simulink model "HL_control_pos_FFforce_RC_WirtualWall_Sync"  (R2020a)
settings: Solver=ode4  StartTime=0.0  StopTime=inf  FixedStep=0.001  RelTol=1e-3
libraries: xpcethercatlib x42, simulink x12, slrtlib x10, AssistOn_Gait_Lib x6
(part 1 of 3)
settings Model: xpc_rtwmakecfg_data=_xpcethercatlib_  SimulationMode=external  Creator=AliYasar  LastModifiedBy=AssistON-Gait
settings DataIOCC: SaveFormat=StructureWithTime
settings OptimizationCC: BlockReduction=off  OptimizeBlockIOStorage=off  BufferReuse=off  GlobalBufferReuse=off  ExpressionFolding=off  LocalBlockOutputs=off  OptimizeDataStoreBuffers=off  BusAssignmentInplaceUpdate=off
settings HardwareCC: ProdBitPerPointer=32  ProdBitPerSizeT=32  ProdBitPerPtrDiffT=32  ProdLargestAtomicFloat=None  ProdWordSize=32  ProdLongLongMode=on  ProdHWDeviceType=Generic->32-bit x86 compatible
settings RTWCC: Description=Simulink Real-Time  SystemTargetFile=slrt.tlc  TemplateMakefile=slrt_default_tmf  CodeExecutionProfiling=on  RTWCompilerOptimization=on
settings SimulinkRealTimeCC: SupportVariableSizeSignals=on  RL32LogTETModifier=off  xPCConcurrentTasks=on  xPCEnableSFAnimation=on

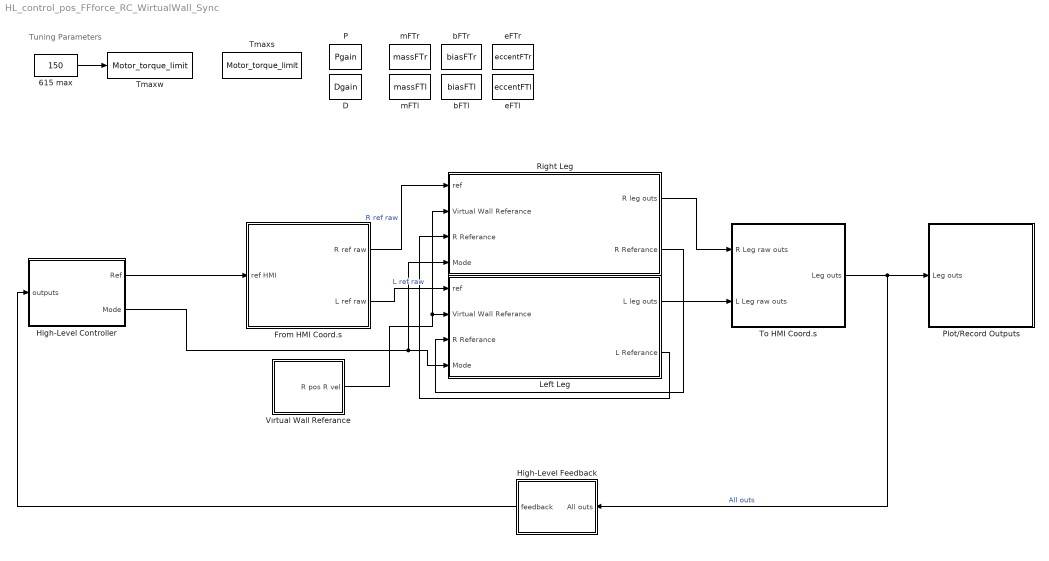
== system HL_control_pos_FFforce_RC_WirtualWall_Sync ==
  note: Tuning Parameters
  615 max : Constant  Value=150
  D : DataStoreMemory  DataStoreName=Dgain  ReadBeforeWriteMsg=warning  WriteAfterWriteMsg=warning  WriteAfterReadMsg=warning  ShowAdditionalParam=off  OutDataTypeStr=double  Dimensions=1
      settings: RTWStateStorageClass=ExportedGlobal
  From HMI Coord.s : Subsystem
  High-Level Controller : Subsystem
  High-Level Feedback : Subsystem
  Left Leg : Subsystem
  P : DataStoreMemory  DataStoreName=Pgain  ReadBeforeWriteMsg=warning  WriteAfterWriteMsg=warning  WriteAfterReadMsg=warning  ShowAdditionalParam=off  OutDataTypeStr=double  Dimensions=1
      settings: RTWStateStorageClass=ExportedGlobal
  Plot/Record Outputs : Subsystem
  Right Leg : Subsystem
  Tmaxs : DataStoreMemory  DataStoreName=Motor_torque_limit  ReadBeforeWriteMsg=warning  WriteAfterWriteMsg=warning  WriteAfterReadMsg=warning  ShowAdditionalParam=off  OutDataTypeStr=double
  Tmaxw : DataStoreWrite  DataStoreName=Motor_torque_limit
  To HMI Coord.s : Subsystem
  Vırtual Wall Referance : Subsystem
  bFTl : DataStoreMemory  DataStoreName=biasFTl  ReadBeforeWriteMsg=warning  WriteAfterWriteMsg=warning  WriteAfterReadMsg=warning  InitialValue=[0; 0; 0; 0; 0; 0]  ShowAdditionalParam=off  OutDataTypeStr=double  Dimensions=[6 1]
      settings: RTWStateStorageClass=ExportedGlobal
  bFTr : DataStoreMemory  DataStoreName=biasFTr  ReadBeforeWriteMsg=warning  WriteAfterWriteMsg=warning  WriteAfterReadMsg=warning  InitialValue=[0; 0; 0; 0; 0; 0]  ShowAdditionalParam=off  OutDataTypeStr=double  Dimensions=[6 1]
      settings: RTWStateStorageClass=ExportedGlobal
  eFTl : DataStoreMemory  DataStoreName=eccentFTl  ReadBeforeWriteMsg=warning  WriteAfterWriteMsg=warning  WriteAfterReadMsg=warning  InitialValue=[0; 0; 0]  ShowAdditionalParam=off  OutDataTypeStr=double  Dimensions=[3 1]
      settings: RTWStateStorageClass=ExportedGlobal
  eFTr : DataStoreMemory  DataStoreName=eccentFTr  ReadBeforeWriteMsg=warning  WriteAfterWriteMsg=warning  WriteAfterReadMsg=warning  InitialValue=[0; 0; 0]  ShowAdditionalParam=off  OutDataTypeStr=double  Dimensions=[3 1]
      settings: RTWStateStorageClass=ExportedGlobal
  mFTl : DataStoreMemory  DataStoreName=massFTl  ReadBeforeWriteMsg=warning  WriteAfterWriteMsg=warning  WriteAfterReadMsg=warning  ShowAdditionalParam=off  OutDataTypeStr=double  Dimensions=1
      settings: RTWStateStorageClass=ExportedGlobal
  mFTr : DataStoreMemory  DataStoreName=massFTr  ReadBeforeWriteMsg=warning  WriteAfterWriteMsg=warning  WriteAfterReadMsg=warning  ShowAdditionalParam=off  OutDataTypeStr=double  Dimensions=1
      settings: RTWStateStorageClass=ExportedGlobal
  wires:
  615 max/1 -> Tmaxw/1
  Left Leg/1(L leg outs) -> To HMI Coord.s/2(L Leg raw outs)
  Right Leg/1(R leg outs) -> To HMI Coord.s/1(R Leg raw outs)
  To HMI Coord.s/1(Leg outs) -> High-Level Feedback/1(All outs), Plot/Record Outputs/1(Leg outs)  "All outs"
  High-Level Controller/1(Ref) -> From HMI Coord.s/1(ref HMI)
  From HMI Coord.s/2(L ref raw) -> Left Leg/1(ref)  "L ref raw"
  From HMI Coord.s/1(R ref raw) -> Right Leg/1(ref)  "R ref raw"
  High-Level Feedback/1(feedback) -> High-Level Controller/1(outputs)
  Right Leg/2(R Referance) -> Left Leg/3(R Referance)
  Left Leg/2(L Referance) -> Right Leg/3("R Referance ")
  Vırtual Wall Referance/1(R pos R vel) -> Left Leg/2(Virtual Wall Referance), Right Leg/2(Virtual Wall Referance)
  High-Level Controller/2(Mode) -> Right Leg/4(Mode), Left Leg/4(Mode)

== system HL_control_pos_FFforce_RC_WirtualWall_Sync/From HMI Coord.s ==
  ref HMI : Inport
  Anti-gravity force : Constant  Value=0
  Bus Selector : BusSelector  OutputSignals=right,left
  "N.m -> mN.m" : Gain  Gain=1000
  Reference : Subsystem
  Subject mass : Constant  Value=0
  Transform L Hip to HMI Coord.s : Subsystem
  Transform R Hip to HMI Coord.s : Subsystem
  R ref raw : Outport
  L ref raw : Outport  Port=2
  wires:
  Transform R Hip to HMI Coord.s/1(R ref raw) -> R ref raw/1  "R ref raw"
  Transform L Hip to HMI Coord.s/1(L ref raw) -> L ref raw/1  "L ref raw"
  Bus Selector/1 -> Transform R Hip to HMI Coord.s/1(R ref HMI)  "<right>"
  Bus Selector/2 -> Transform L Hip to HMI Coord.s/2(L ref HMI)  "<left>"
  Subject mass/1 -> "N.m -> mN.m"/1
  ref HMI/1 -> Reference/1(HMI ref), Bus Selector/1  "HMI ref"
  "N.m -> mN.m"/1 -> Transform L Hip to HMI Coord.s/1(T scale), Transform R Hip to HMI Coord.s/2(T scale)
  Anti-gravity force/1 -> Transform L Hip to HMI Coord.s/3(In3), Transform R Hip to HMI Coord.s/3(In3)

== system HL_control_pos_FFforce_RC_WirtualWall_Sync/High-Level Controller ==
  outputs : Inport
  Home Position: 0 Calibration: 1 Force Control w/ FSR: 2 Power OFF: any : Constant  Value=0
  Reference Generator : Stateflow chart  TreatAsAtomicUnit=on
      settings: PortSchema="{\"entries\":[{\"content\":{\"sides\":[{\"content\":{\"connectorIds\":[\"In1\",\"In4\",\"In2\",\"In3\"]},\"type\":\"ConnectorPlacement.EquallySpacedRectSide\",\"uuid\":\"aa4ba9cf-5d9b-4aac-b6bf-f3c223218dd1\"},{\"content\":{\"connectorIds\":[\"Out1\"],\"side\":\"RIGHT\"},\"type\":\"ConnectorPlacement.EquallySpacedRectSide\",\"uuid\":\"cd1fa299-8856-4d1c-b1a3-02aa84ed53a9\"},{\"content\":{\"connectorIds\":[\"In5\"],\"side\":\"TOP\"},\"type\":\"ConnectorPlacement.EquallySpacedRectSide\",\"uuid\":\"78c29b93-9a46-49f0-9d97-93372759fd65\"}]},\"type\":\"ConnectorPlacement.EquallySpacedConnector\",\"uuid\":\"ad73f022-92f1-404d-a46a-c53ca5f2e508\"}],\"packageUris\":[\"http://schema.mathworks.com/mf0/Connector/19700101\"],\"version\":\"1.0\"}"
  Select outputs : Subsystem
  System Enable : Stateflow chart  TreatAsAtomicUnit=on
      settings: PortSchema="{\"entries\":[{\"content\":{\"sides\":[{\"content\":{\"connectorIds\":[\"In2\",\"In1\"]},\"type\":\"ConnectorPlacement.EquallySpacedRectSide\",\"uuid\":\"4b9d4f11-1327-467a-8cb8-f29f037cc139\"},{\"content\":{\"connectorIds\":[\"Out2\",\"Out1\"],\"side\":\"RIGHT\"},\"type\":\"ConnectorPlacement.EquallySpacedRectSide\",\"uuid\":\"fda62fdb-ec88-4c1e-8450-5399b215f716\"},{\"content\":{\"connectorIds\":[],\"side\":\"TOP\"},\"type\":\"ConnectorPlacement.EquallySpacedRectSide\",\"uuid\":\"5cb4c28a-5e87-4a76-a578-be8042483ab0\"}]},\"type\":\"ConnectorPlacement.EquallySpacedConnector\",\"uuid\":\"90f57a99-7211-48b6-a431-558685cd5a2d\"}],\"packageUris\":[\"http://schema.mathworks.com/mf0/Connector/19700101\"],\"version\":\"1.0\"}"
  "To clear the error, change the value to any number" : Constant
  Ref : Outport
  Mode : Outport  Port=2
  tag scope: status=global
  wires:
  Reference Generator/1(ref) -> Ref/1  "HMI ref"
  System Enable/1(sysON) -> Reference Generator/1(sysON)
  Home Position: 0 Calibration: 1 Force Control w/ FSR: 2 Power OFF: any/1 -> Reference Generator/5(MODE), Mode/1
  "To clear the error, change the value to any number"/1 -> System Enable/2(clear)
  outputs/1 -> Select outputs/1(outs)
  Select outputs/1(disk angles) -> System Enable/1(diskpos)
  Select outputs/2(gait out) -> Reference Generator/4(gait)
  Select outputs/3(FT out) -> Reference Generator/2(FT)
  Select outputs/4(EE mot) -> Reference Generator/3(mot)
  System Enable/2(stat) -> [status]

== system HL_control_pos_FFforce_RC_WirtualWall_Sync/High-Level Feedback ==
  All outs : Inport
  Bus Creator : BusCreator  Inputs=3
  Bus Creator1 : BusCreator  Inputs=2  OutDataTypeStr=Bus: HeelForce
      settings: InheritFromInputs=off
  Bus Selector : BusSelector  OutputSignals=R Leg outs.R_foot_sens,L Leg outs.L_foot_sens,R Leg outs,L Leg outs
  Heel Sensor : Stateflow chart  TreatAsAtomicUnit=on
  feedback : Outport
  wires:
  Bus Creator/1 -> feedback/1
  Heel Sensor/1(gait) -> Bus Creator/1
  Bus Selector/2 -> Bus Creator1/2  "<L_foot_sens>"
  Bus Selector/4 -> Bus Creator/3  "<L Leg outs>"
  Bus Creator1/1 -> Heel Sensor/1(heel_force)
  Bus Selector/1 -> Bus Creator1/1  "<R_foot_sens>"
  Bus Selector/3 -> Bus Creator/2  "<R Leg outs>"
  All outs/1 -> Bus Selector/1

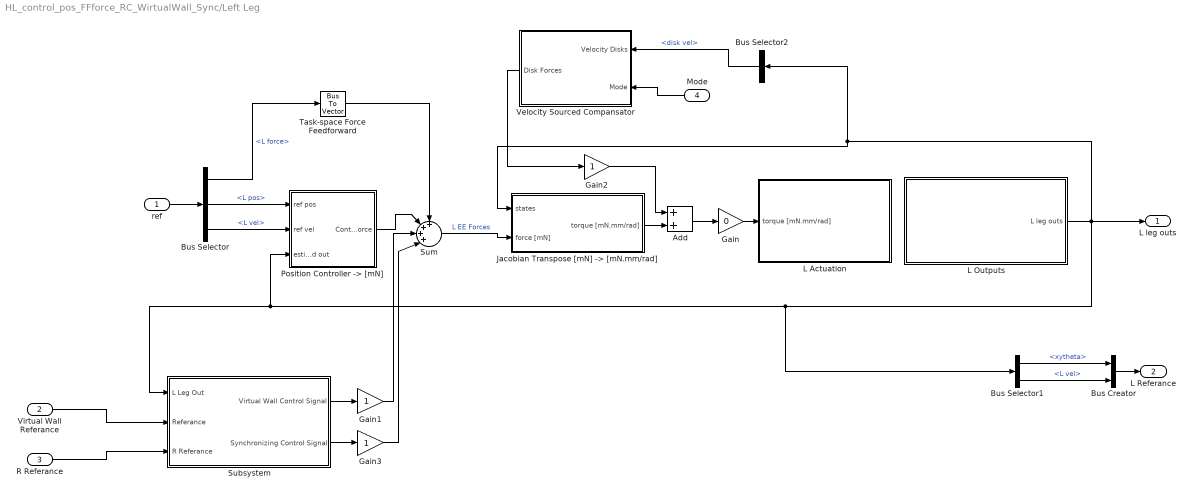
== system HL_control_pos_FFforce_RC_WirtualWall_Sync/Left Leg ==
  ref : Inport
  Virtual Wall Referance : Inport  Port=2
  R Referance : Inport  Port=3
  Mode : Inport  Port=4
  Add : Sum
  Bus Creator : BusCreator  Inputs=2
  Bus Selector : BusSelector  OutputSignals=L force,L pos,L vel
  Bus Selector1 : BusSelector  OutputSignals=L pos.xytheta,L vel
  Bus Selector2 : BusSelector  OutputSignals=L disk mot.disk vel
  Gain : Gain  Gain=0
  Gain1 : Gain
  Gain2 : Gain
  Gain3 : Gain
  "Jacobian Transpose [mN] -> [mN.mm/rad]" : Subsystem
  L Actuation : Subsystem
  L Outputs : Subsystem
  "Position Controller -> [mN]" : Subsystem
  Subsystem : Subsystem
  Sum : Sum  Inputs=++++|
  Task-space Force Feedforward : BusToVector
  Velocity Sourced Compansator : Subsystem
  L leg outs : Outport
  L Referance : Outport  Port=2
  wires:
  Task-space Force Feedforward/1 -> Sum/1
  Gain/1 -> L Actuation/1(torque [mN.mm/rad])
  ref/1 -> Bus Selector/1
  Bus Selector/2 -> "Position Controller -> [mN]"/1(ref pos)  "<L pos>"
  Bus Selector/1 -> Task-space Force Feedforward/1  "<L force>"
  "Position Controller -> [mN]"/1(Control Force) -> Sum/2
  Sum/1 -> "Jacobian Transpose [mN] -> [mN.mm/rad]"/2(force [mN])  "L EE Forces"
  Bus Selector/3 -> "Position Controller -> [mN]"/2(ref vel)  "<L vel>"
  Bus Selector1/1 -> Bus Creator/1  "<xytheta>"
  Bus Selector1/2 -> Bus Creator/2  "<L vel>"
  Bus Creator/1 -> L Referance/1
  L Outputs/1(L leg outs) -> Bus Selector1/1, Subsystem/1(L Leg Out), "Position Controller -> [mN]"/3(estimated out), Bus Selector2/1, "Jacobian Transpose [mN] -> [mN.mm/rad]"/1(states), L leg outs/1
  Mode/1 -> Velocity Sourced Compansator/2(Mode)
  Bus Selector2/1 -> Velocity Sourced Compansator/1(Velocity Disks)  "<disk vel>"
  "Jacobian Transpose [mN] -> [mN.mm/rad]"/1(torque [mN.mm/rad]) -> Add/2
  Add/1 -> Gain/1
  Velocity Sourced Compansator/1(Disk Forces) -> Gain2/1
  Gain2/1 -> Add/1
  Virtual Wall Referance/1 -> Subsystem/2(Referance)
  R Referance/1 -> Subsystem/3(R Referance)
  Subsystem/1(Virtual Wall Control Signal) -> Gain1/1
  Subsystem/2(Synchronizing Control Signal) -> Gain3/1
  Gain1/1 -> Sum/3
  Gain3/1 -> Sum/4

== system HL_control_pos_FFforce_RC_WirtualWall_Sync/Plot//Record Outputs ==
  Leg outs : Inport
  Bus Creator2 : BusCreator  Inputs=3
  Bus Selector1 : BusSelector  OutputSignals=R Leg outs.rFT.rFx,R Leg outs.rFT.rFy,R Leg outs.rFT.rTx,R Leg outs.rFT.rTy,R Leg outs.rFT.rTz,L Leg outs.lFT.lFx,L Leg outs.lFT.lFy,L Leg outs.lFT.lTx,L Leg outs.lFT.lTy,L Leg outs.lFT.lTz  OutputAsBus=on
  Bus Selector3 : BusSelector  OutputSignals=R Leg outs.R Motor Torques,L Leg outs.L Motor Torques  OutputAsBus=on
  Bus Selector4 : BusSelector  OutputSignals=R Leg outs.R_foot_sens,L Leg outs.L_foot_sens  OutputAsBus=on
  Bus Selector5 : BusSelector  OutputSignals=R Leg outs,L Leg outs
  FT Readings : slrtlib/Displays and Logging/Scope   scopeno=12  scopetype=Target  autostart=on  viewmode=Numerical  formatstr='%15.6f'  grid=on  ylimits=100*[-1, 1]  nosamples=10  noprepostsamples=0  interleave=10  triggermode=FreeRun  triggersignal=1  trigsignalfromport=off  triggerlevel=0.0  triggerslope=Either  triggerscope=1  triggersample=0  filename=data.dat  mode=Lazy  writesize=512  autorestart=off  dynamicfilemode=off  maxwritefilesize=512*1024^2
  Heel Strikes : slrtlib/Displays and Logging/Scope   scopeno=13  scopetype=Target  autostart=on  viewmode=Graphical rolling  formatstr='%15.6f'  grid=on  ylimits=5*[-0.2, 1]  nosamples=500  noprepostsamples=0  interleave=20  triggermode=FreeRun  triggersignal=1  trigsignalfromport=off  triggerlevel=0.0  triggerslope=Either  triggerscope=1  triggersample=0  filename=data.dat  mode=Lazy  writesize=512  autorestart=off  dynamicfilemode=off  maxwritefilesize=512*1024^2
  Left leg readings : Subsystem
  Motor Torque Demand : slrtlib/Displays and Logging/Scope   scopeno=11  scopetype=Target  autostart=on  viewmode=Numerical  formatstr='%15.6f'  grid=on  ylimits=100*[-1, 1]  nosamples=10  noprepostsamples=0  interleave=10  triggermode=FreeRun  triggersignal=1  trigsignalfromport=off  triggerlevel=0.0  triggerslope=Either  triggerscope=1  triggersample=0  filename=data.dat  mode=Lazy  writesize=512  autorestart=off  dynamicfilemode=off  maxwritefilesize=512*1024^2
  Right leg readings : Subsystem
  "Scope " : slrtlib/Displays and Logging/Scope   scopeno=100  scopetype=File  autostart=on  viewmode=Numerical  formatstr='%15.6f'  grid=on  ylimits=[0,0]  nosamples=100*60*60  noprepostsamples=0  interleave=10  triggermode=FreeRun  triggersignal=1  trigsignalfromport=off  triggerlevel=0.0  triggerslope=Either  triggerscope=1  triggersample=0  filename=alldata.dat  mode=Lazy  writesize=512  autorestart=off  dynamicfilemode=off  maxwritefilesize=512*1024^2
  wires:
  Bus Creator2/1 -> "Scope "/1
  Bus Selector3/1 -> Motor Torque Demand/1
  [Ref] -> Bus Creator2/2  "HMI ref"
  Bus Selector1/1 -> FT Readings/1
  Bus Selector5/2 -> Left leg readings/1(L outs)  "<L Leg outs>"
  Leg outs/1 -> Bus Selector5/1, Bus Creator2/1, Bus Selector3/1, Bus Selector4/1, Bus Selector1/1
  Bus Selector5/1 -> Right leg readings/1(R outs)  "<R Leg outs>"
  Bus Selector4/1 -> Heel Strikes/1
  [status] -> Bus Creator2/3

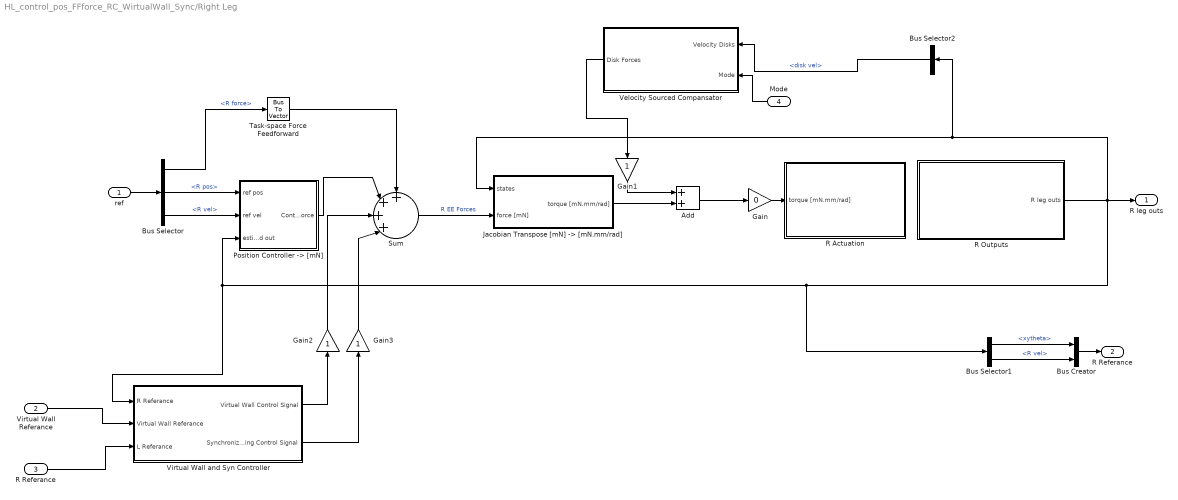
== system HL_control_pos_FFforce_RC_WirtualWall_Sync/Right Leg ==
  ref : Inport
  Virtual Wall Referance : Inport  Port=2
  "R Referance " : Inport  Port=3
  Mode : Inport  Port=4
  Add : Sum
  Bus Creator : BusCreator  Inputs=2
  Bus Selector : BusSelector  OutputSignals=R force,R pos,R vel
  Bus Selector1 : BusSelector  OutputSignals=R pos.xytheta,R vel
  Bus Selector2 : BusSelector  OutputSignals=R disk mot.disk vel
  Gain : Gain  Gain=0
  Gain1 : Gain
  Gain2 : Gain
  Gain3 : Gain
  "Jacobian Transpose [mN] -> [mN.mm/rad]" : Subsystem
  "Position Controller -> [mN]" : Subsystem
  R Actuation : Subsystem
  R Outputs : Subsystem
  Sum : Sum  Inputs=++++|
  Task-space Force Feedforward : BusToVector
  Velocity Sourced Compansator : Subsystem
  Virtual Wall and Syn Controller : Subsystem
  R leg outs : Outport
  R Referance : Outport  Port=2
  wires:
  Gain/1 -> R Actuation/1(torque [mN.mm/rad])
  Bus Selector/1 -> Task-space Force Feedforward/1  "<R force>"
  ref/1 -> Bus Selector/1
  Bus Selector/2 -> "Position Controller -> [mN]"/1(ref pos)  "<R pos>"
  Sum/1 -> "Jacobian Transpose [mN] -> [mN.mm/rad]"/2(force [mN])  "R EE Forces"
  Bus Selector/3 -> "Position Controller -> [mN]"/2(ref vel)  "<R vel>"
  Bus Creator/1 -> R Referance/1
  Bus Selector1/1 -> Bus Creator/1  "<xytheta>"
  Bus Selector1/2 -> Bus Creator/2  "<R vel>"
  R Outputs/1(R leg outs) -> Bus Selector1/1, Virtual Wall and Syn Controller/1(R Referance), "Position Controller -> [mN]"/3(estimated out), R leg outs/1, "Jacobian Transpose [mN] -> [mN.mm/rad]"/1(states), Bus Selector2/1
  Bus Selector2/1 -> Velocity Sourced Compansator/1(Velocity Disks)  "<disk vel>"
  Mode/1 -> Velocity Sourced Compansator/2(Mode)
  Task-space Force Feedforward/1 -> Sum/1
  "Position Controller -> [mN]"/1(Control Force) -> Sum/2
  "Jacobian Transpose [mN] -> [mN.mm/rad]"/1(torque [mN.mm/rad]) -> Add/2
  Add/1 -> Gain/1
  Velocity Sourced Compansator/1(Disk Forces) -> Gain1/1
  Virtual Wall Referance/1 -> Virtual Wall and Syn Controller/2(Virtual Wall Referance)
  "R Referance "/1 -> Virtual Wall and Syn Controller/3(L Referance)
  Virtual Wall and Syn Controller/1(Virtual Wall Control Signal) -> Gain2/1
  Virtual Wall and Syn Controller/2(Synchronizing Control Signal) -> Gain3/1
  Gain1/1 -> Add/1
  Gain2/1 -> Sum/3
  Gain3/1 -> Sum/4

== system HL_control_pos_FFforce_RC_WirtualWall_Sync/To HMI Coord.s ==
  R Leg raw outs : Inport
  L Leg raw outs : Inport  Port=2
  Bus Creator : BusCreator  Inputs=7
  Bus Creator1 : BusCreator  Inputs=2
  Bus Creator2 : BusCreator  Inputs=7
  Bus Selector : BusSelector  OutputSignals=R pos.xytheta,R vel,R_thigh_FT,R disk mot,R_foot_sens,R Motor Torques,R disk torque
  Bus Selector1 : BusSelector  OutputSignals=L pos.xytheta,L vel,L_thigh_FT,L disk mot,L_foot_sens,L Motor Torques,L disk torque
  L Leg : Subsystem
  R Leg : Subsystem
  Leg outs : Outport
  wires:
  R Leg/1(R pos) -> Bus Creator/1  "rpos"
  R Leg/2(R vel) -> Bus Creator/2  "rvel"
  R Leg raw outs/1 -> Bus Selector/1
  Bus Selector/1 -> R Leg/1(pos)  "<xytheta>"
  Bus Selector/2 -> R Leg/2(vel)  "<R vel>"
  Bus Selector1/2 -> L Leg/2(vel)  "<L vel>"
  Bus Selector1/1 -> L Leg/1(pos)  "<xytheta>"
  L Leg raw outs/1 -> Bus Selector1/1
  Bus Creator/1 -> Bus Creator1/1  "R Leg outs"
  L Leg/2(L vel) -> Bus Creator2/2  "lvel"
  L Leg/1(L pos) -> Bus Creator2/1  "lpos"
  Bus Selector/4 -> Bus Creator/4  "<R disk mot>"
  Bus Selector/5 -> Bus Creator/5  "<R_foot_sens>"
  Bus Creator2/1 -> Bus Creator1/2  "L Leg outs"
  Bus Selector1/4 -> Bus Creator2/4  "<L disk mot>"
  Bus Selector1/5 -> Bus Creator2/5  "<L_foot_sens>"
  Bus Selector/3 -> R Leg/3(FT)  "<R_thigh_FT>"
  Bus Selector1/3 -> L Leg/3(FT)  "<L_thigh_FT>"
  R Leg/3(R FT) -> Bus Creator/3  "rFT"
  L Leg/3(L FT) -> Bus Creator2/3  "lFT"
  Bus Selector/6 -> Bus Creator/6  "<R Motor Torques>"
  Bus Selector1/6 -> Bus Creator2/6  "<L Motor Torques>"
  Bus Creator1/1 -> Leg outs/1
  Bus Selector/7 -> Bus Creator/7  "<R disk torque>"
  Bus Selector1/7 -> Bus Creator2/7  "<L disk torque>"

== system HL_control_pos_FFforce_RC_WirtualWall_Sync/Vırtual Wall Referance ==
  Bus Creator : BusCreator  Inputs=2
  Constant : Constant  Value=[0,0,0]
  Constant1 : Constant  Value=[0,0,0]
  Demux : Demux  Outputs=3
  Demux1 : Demux  Outputs=3
  MATLAB Function : MATLAB Function  TreatAsAtomicUnit=on
  Terminator{,1..3} (4 alike) : Terminator
  R pos R vel : Outport
  wires:
  Constant/1 -> MATLAB Function/1("pos ")
  Constant1/1 -> MATLAB Function/2("vel ")
  Bus Creator/1 -> R pos R vel/1
  MATLAB Function/1(pos) -> Demux/1
  Demux/1 -> Bus Creator/1  "X"
  MATLAB Function/2(vel) -> Demux1/1
  Demux/2 -> Terminator1/1
  Demux/3 -> Terminator/1
  Demux1/3 -> Terminator2/1
  Demux1/2 -> Terminator3/1
  Demux1/1 -> Bus Creator/2  "Xdot"

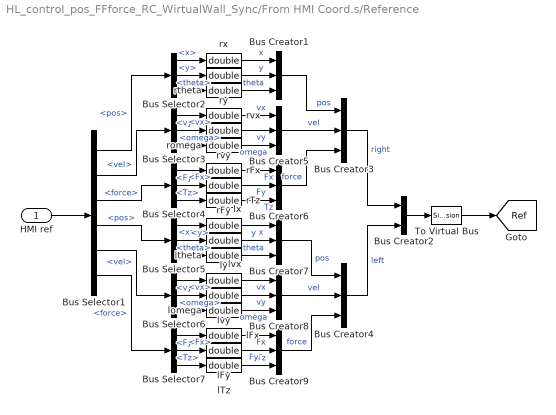
== system HL_control_pos_FFforce_RC_WirtualWall_Sync/From HMI Coord.s/Reference ==
  HMI ref : Inport
  Bus Creator{1,3..9} (8 alike) : BusCreator  Inputs=3
  Bus Creator2 : BusCreator  Inputs=2
  Bus Selector1 : BusSelector  OutputSignals=right.pos,right.vel,right.force,left.pos,left.vel,left.force
  Bus Selector2 : BusSelector  OutputSignals=x,y,theta
  Bus Selector3 : BusSelector  OutputSignals=vx,vy,omega
  Bus Selector4 : BusSelector  OutputSignals=Fx,Fy,Tz
  Bus Selector5 : BusSelector  OutputSignals=x,y,theta
  Bus Selector6 : BusSelector  OutputSignals=vx,vy,omega
  Bus Selector7 : BusSelector  OutputSignals=Fx,Fy,Tz
  To Virtual Bus : SignalConversion  ConversionOutput=Virtual bus  OverrideOpt=off
  lFx : DataTypeConversion  OutDataTypeStr=double
  lFy : DataTypeConversion  OutDataTypeStr=double
  lTz : DataTypeConversion  OutDataTypeStr=double
  lomega : DataTypeConversion  OutDataTypeStr=double
  ltheta : DataTypeConversion  OutDataTypeStr=double
  lvx : DataTypeConversion  OutDataTypeStr=double
  lvy : DataTypeConversion  OutDataTypeStr=double
  lx : DataTypeConversion  OutDataTypeStr=double
  ly : DataTypeConversion  OutDataTypeStr=double
  rFx : DataTypeConversion  OutDataTypeStr=double
  rFy : DataTypeConversion  OutDataTypeStr=double
  rTz : DataTypeConversion  OutDataTypeStr=double
  romega : DataTypeConversion  OutDataTypeStr=double
  rtheta : DataTypeConversion  OutDataTypeStr=double
  rvx : DataTypeConversion  OutDataTypeStr=double
  rvy : DataTypeConversion  OutDataTypeStr=double
  rx : DataTypeConversion  OutDataTypeStr=double
  ry : DataTypeConversion  OutDataTypeStr=double
  tag scope: Ref=global
  wires:
  Bus Selector3/2 -> rvy/1  "<vy>"
  To Virtual Bus/1 -> [Ref]
  Bus Selector2/1 -> rx/1  "<x>"
  romega/1 -> Bus Creator5/3  "omega"
  Bus Creator7/1 -> Bus Creator4/1  "pos"
  rvx/1 -> Bus Creator5/1  "vx"
  Bus Selector3/1 -> rvx/1  "<vx>"
  Bus Selector3/3 -> romega/1  "<omega>"
  Bus Selector1/4 -> Bus Selector5/1  "<pos>"
  Bus Creator2/1 -> To Virtual Bus/1
  ry/1 -> Bus Creator1/2  "y"
  rvy/1 -> Bus Creator5/2  "vy"
  Bus Selector4/2 -> rFy/1  "<Fy>"
  Bus Creator3/1 -> Bus Creator2/1  "right"
  Bus Selector6/2 -> lvy/1  "<vy>"
  Bus Selector4/3 -> rTz/1  "<Tz>"
  Bus Selector6/1 -> lvx/1  "<vx>"
  Bus Creator4/1 -> Bus Creator2/2  "left"
  Bus Creator1/1 -> Bus Creator3/1  "pos"
  Bus Selector1/1 -> Bus Selector2/1  "<pos>"
  lvx/1 -> Bus Creator8/1  "vx"
  Bus Selector1/2 -> Bus Selector3/1  "<vel>"
  Bus Selector2/3 -> rtheta/1  "<theta>"
  rtheta/1 -> Bus Creator1/3  "theta"
  ltheta/1 -> Bus Creator7/3  "theta"
  Bus Creator9/1 -> Bus Creator4/3  "force"
  Bus Selector2/2 -> ry/1  "<y>"
  Bus Selector5/3 -> ltheta/1  "<theta>"
  lFx/1 -> Bus Creator9/1  "Fx"
  rx/1 -> Bus Creator1/1  "x"
  Bus Selector1/6 -> Bus Selector7/1  "<force>"
  Bus Selector5/1 -> lx/1  "<x>"
  Bus Selector4/1 -> rFx/1  "<Fx>"
  Bus Selector1/5 -> Bus Selector6/1  "<vel>"
  Bus Selector1/3 -> Bus Selector4/1  "<force>"
  rFx/1 -> Bus Creator6/1  "Fx"
  rFy/1 -> Bus Creator6/2  "Fy"
  rTz/1 -> Bus Creator6/3  "Tz"
  Bus Creator5/1 -> Bus Creator3/2  "vel"
  lTz/1 -> Bus Creator9/3  "Tz"
  Bus Selector7/2 -> lFy/1  "<Fy>"
  lvy/1 -> Bus Creator8/2  "vy"
  Bus Selector7/1 -> lFx/1  "<Fx>"
  Bus Creator8/1 -> Bus Creator4/2  "vel"
  Bus Selector7/3 -> lTz/1  "<Tz>"
  Bus Selector5/2 -> ly/1  "<y>"
  lFy/1 -> Bus Creator9/2  "Fy"
  Bus Selector6/3 -> lomega/1  "<omega>"
  lomega/1 -> Bus Creator8/3  "omega"
  lx/1 -> Bus Creator7/1  "x"
  ly/1 -> Bus Creator7/2  "y"
  Bus Creator6/1 -> Bus Creator3/3  "force"
  HMI ref/1 -> Bus Selector1/1

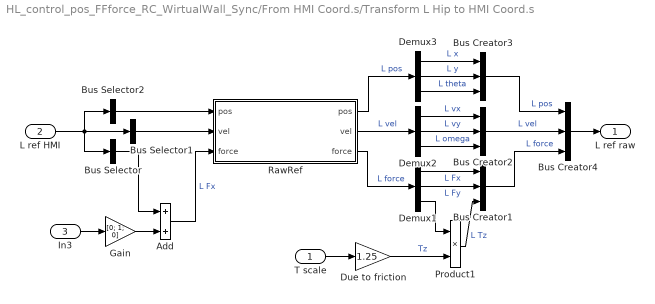
== system HL_control_pos_FFforce_RC_WirtualWall_Sync/From HMI Coord.s/Transform L Hip to HMI Coord.s ==
  T scale : Inport
  L ref HMI : Inport  Port=2
  In3 : Inport  Port=3
  Add : Sum
  Bus Creator{1..4} (4 alike) : BusCreator  Inputs=3
  Bus Selector : BusSelector  OutputSignals=force.Fx,force.Fy,force.Tz  OutputAsBus=on
  Bus Selector1 : BusSelector  OutputSignals=vel.vx,vel.vy,vel.omega  OutputAsBus=on
  Bus Selector2 : BusSelector  OutputSignals=pos.x,pos.y,pos.theta  OutputAsBus=on
  Demux1 : Demux  Outputs=3
  Demux2 : Demux  Outputs=3
  Demux3 : Demux  Outputs=3
  Due to friction : Gain  Gain=1.25
  Gain : Gain  Gain=[0; 1; 0]
  Product1 : Product  OutDataTypeStr=Inherit: Inherit via back propagation
  RawRef : MATLAB Function  TreatAsAtomicUnit=on
  L ref raw : Outport
  wires:
  T scale/1 -> Due to friction/1
  Due to friction/1 -> Product1/2  "Tz"
  Product1/1 -> Bus Creator1/3  "L Tz"
  Demux1/3 -> Product1/1
  Demux2/1 -> Bus Creator2/1  "L vx"
  Demux2/2 -> Bus Creator2/2  "L vy"
  Demux2/3 -> Bus Creator2/3  "L omega"
  Demux3/2 -> Bus Creator3/2  "L y"
  Bus Creator2/1 -> Bus Creator4/2  "L vel"
  Demux1/1 -> Bus Creator1/1  "L Fx"
  RawRef/1(pos) -> Demux3/1  "L pos"
  Demux1/2 -> Bus Creator1/2  "L Fy"
  RawRef/3(force) -> Demux1/1  "L force"
  Demux3/3 -> Bus Creator3/3  "L theta"
  Bus Creator1/1 -> Bus Creator4/3  "L force"
  Demux3/1 -> Bus Creator3/1  "L x"
  Bus Creator3/1 -> Bus Creator4/1  "L pos"
  Bus Creator4/1 -> L ref raw/1
  RawRef/2(vel) -> Demux2/1  "L vel"
  L ref HMI/1 -> Bus Selector2/1, Bus Selector1/1, Bus Selector/1
  Bus Selector1/1 -> RawRef/2("vel ")
  Bus Selector2/1 -> RawRef/1("pos ")
  Bus Selector/1 -> Add/1
  Gain/1 -> Add/2
  In3/1 -> Gain/1
  Add/1 -> RawRef/3("force ")  "L Fx"

== system HL_control_pos_FFforce_RC_WirtualWall_Sync/From HMI Coord.s/Transform R Hip to HMI Coord.s ==
  R ref HMI : Inport
  T scale : Inport  Port=2
  In3 : Inport  Port=3
  Add : Sum
  Bus Creator{,1..3} (4 alike) : BusCreator  Inputs=3
  Bus Selector : BusSelector  OutputSignals=force.Fx,force.Fy,force.Tz  OutputAsBus=on
  Bus Selector1 : BusSelector  OutputSignals=vel.vx,vel.vy,vel.omega  OutputAsBus=on
  Bus Selector2 : BusSelector  OutputSignals=pos.x,pos.y,pos.theta  OutputAsBus=on
  Demux : Demux  Outputs=3
  Demux1 : Demux  Outputs=3
  Demux2 : Demux  Outputs=3
  Gain : Gain  Gain=[0; 1; 0]
  Product : Product  OutDataTypeStr=Inherit: Inherit via back propagation
  RawRef : MATLAB Function  TreatAsAtomicUnit=on
  R ref raw : Outport
  wires:
  RawRef/3(force) -> Demux/1  "R force"
  R ref HMI/1 -> Bus Selector2/1, Bus Selector1/1, Bus Selector/1
  Demux/1 -> Bus Creator/1  "R Fx"
  Demux/2 -> Bus Creator/2  "R Fy"
  Product/1 -> Bus Creator/3  "R Tz"
  Bus Creator/1 -> Bus Creator3/3  "R force"
  Bus Creator1/1 -> Bus Creator3/2  "R vel"
  Demux1/3 -> Bus Creator1/3  "R omega"
  Demux1/2 -> Bus Creator1/2  "R vy"
  Demux1/1 -> Bus Creator1/1  "R vx"
  RawRef/2(vel) -> Demux1/1  "R vel"
  RawRef/1(pos) -> Demux2/1  "R pos"
  Demux2/1 -> Bus Creator2/1  "R x"
  Demux2/2 -> Bus Creator2/2  "R y"
  Demux2/3 -> Bus Creator2/3  "R theta"
  Bus Creator2/1 -> Bus Creator3/1  "R pos"
  Bus Creator3/1 -> R ref raw/1
  Bus Selector/1 -> Add/1
  T scale/1 -> Product/2
  Demux/3 -> Product/1
  Bus Selector2/1 -> RawRef/1("pos ")
  Bus Selector1/1 -> RawRef/2("vel ")
  In3/1 -> Gain/1
  Gain/1 -> Add/2
  Add/1 -> RawRef/3("force ")  "R Fx"

== system HL_control_pos_FFforce_RC_WirtualWall_Sync/High-Level Controller/Reference Generator/SystemON.ForceTrajectoryGeneretor.DataHandling.ReadData.read_data ==
  f : TriggerPort  TriggerType=function-call  VariantControl=(inherit)  SampleTime=0.001
      settings: CopyFcn=Stateflow.SLINSF.SimulinkMan.removeBlockPreDeleteFcn  PreDeleteFcn=Stateflow.SLINSF.SimulinkMan.unsafePredeleteFcn
  From File : FromFile  FileName=hip_moment.mat
  force : Outport
  wires:
  From File/1 -> force/1

== system HL_control_pos_FFforce_RC_WirtualWall_Sync/High-Level Controller/Reference Generator/SystemON.ForceTrajectoryGeneretor.getCustomTrajectory ==
  f : TriggerPort  TriggerType=function-call  VariantControl=(inherit)  SampleTimeType=periodic  SampleTime=0.001
      settings: CopyFcn=Stateflow.SLINSF.SimulinkMan.removeBlockPreDeleteFcn  PreDeleteFcn=Stateflow.SLINSF.SimulinkMan.unsafePredeleteFcn
  Bus Creator3 : BusCreator  Commented=on  Inputs=3  OutDataTypeStr=Bus: Force
  Fx : Sin  Commented=on  Amplitude=20*0  Frequency=0.5  Phase=pi/2  SampleTime=0.001
  Fy : Sin  Commented=on  Amplitude=20*0  Frequency=0.5  SampleTime=0.001
  Tz : Sin  Commented=on  Amplitude=0  Frequency=2  Phase=pi  SampleTime=0.001
  force : Outport
  wires:
  Fy/1 -> Bus Creator3/2  "Fy"
  Tz/1 -> Bus Creator3/3  "Tz"
  Fx/1 -> Bus Creator3/1  "Fx"
  Bus Creator3/1 -> force/1  "ref"

== system HL_control_pos_FFforce_RC_WirtualWall_Sync/High-Level Controller/Reference Generator/SystemON.MotionTrajectoryGenerator.Calibration.read_data ==
  f : TriggerPort  TriggerType=function-call  VariantControl=(inherit)  SampleTime=0.001
      settings: CopyFcn=Stateflow.SLINSF.SimulinkMan.removeBlockPreDeleteFcn  PreDeleteFcn=Stateflow.SLINSF.SimulinkMan.unsafePredeleteFcn
  From File : FromFile  FileName=calib_pos.mat
  From File1 : FromFile  FileName=calib_vel.mat
  Vector Concatenate : Concatenate  Mode=Multidimensional array  ConcatenateDimension=2
  cmot : Outport
  wires:
  From File/1 -> Vector Concatenate/1
  From File1/1 -> Vector Concatenate/2
  Vector Concatenate/1 -> cmot/1

== system HL_control_pos_FFforce_RC_WirtualWall_Sync/High-Level Controller/Reference Generator/SystemON.MotionTrajectoryGenerator.testTrajectory ==
  f : TriggerPort  TriggerType=function-call  VariantControl=(inherit)  SampleTimeType=periodic  SampleTime=0.001
      settings: CopyFcn=Stateflow.SLINSF.SimulinkMan.removeBlockPreDeleteFcn  PreDeleteFcn=Stateflow.SLINSF.SimulinkMan.unsafePredeleteFcn
  Bus Creator : BusCreator  Inputs=3  OutDataTypeStr=Bus: Pos
      settings: InheritFromInputs=off
  Bus Creator1 : BusCreator  Inputs=3  OutDataTypeStr=Bus: Vel
      settings: InheritFromInputs=off
  Bus to Vector : BusToVector
  Bus to Vector1 : BusToVector
  Cast To Double : DataTypeConversion  OutDataTypeStr=double
  Cast To Double1 : DataTypeConversion  OutDataTypeStr=double
  theta : Sin  Amplitude=pi/5  Frequency=1.5  SampleTime=0.001
  thetad : Sin  Amplitude=pi/5*1.5  Frequency=1.5  Phase=pi/2  SampleTime=0.001
  x : Sin  Amplitude=20  Frequency=1.5  Phase=pi/2  SampleTime=0.001
  xd : Sin  Amplitude=20*1.5  Frequency=1.5  Phase=pi  SampleTime=0.001
  y : Sin  Amplitude=20  Frequency=1.5  SampleTime=0.001
  yd : Sin  Amplitude=20*1.5  Frequency=1.5  Phase=pi/2  SampleTime=0.001
  pos : Outport
  vel : Outport  Port=2
  wires:
  Bus Creator/1 -> Bus to Vector/1
  Bus Creator1/1 -> Bus to Vector1/1
  Bus to Vector/1 -> Cast To Double/1
  Bus to Vector1/1 -> Cast To Double1/1
  y/1 -> Bus Creator/2  "ref y"
  theta/1 -> Bus Creator/3  "ref theta"
  x/1 -> Bus Creator/1  "ref x"
  yd/1 -> Bus Creator1/2  "ref vy"
  thetad/1 -> Bus Creator1/3  "ref omega"
  xd/1 -> Bus Creator1/1  "ref vx"
  Cast To Double/1 -> pos/1
  Cast To Double1/1 -> vel/1

== system HL_control_pos_FFforce_RC_WirtualWall_Sync/High-Level Controller/Reference Generator/SystemON.setControl1 ==
  c : Inport  OutDataTypeStr=double  PortDimensions=1
  f : TriggerPort  TriggerType=function-call  VariantControl=(inherit)  SampleTimeType=periodic  SampleTime=0.001
      settings: CopyFcn=Stateflow.SLINSF.SimulinkMan.removeBlockPreDeleteFcn  PreDeleteFcn=Stateflow.SLINSF.SimulinkMan.unsafePredeleteFcn
  Data Type Conversion : DataTypeConversion  OutDataTypeStr=uint32
  "EtherCAT PDO Transmit " : xpcethercatlib/EtherCAT PDO Transmit   Priority=3  sig_name=Right F/T.Control Codes.Control 1  sig_offset=576  sig_type=uint32  type_size=32  sig_dim=1  device_id=0  sample_time=0.001000
      settings: SourceProductBaseCode=XP
  EtherCAT PDO Transmit 1 : xpcethercatlib/EtherCAT PDO Transmit   Priority=3  sig_name=Left F/T.Control Codes.Control 1  sig_offset=1536  sig_type=uint32  type_size=32  sig_dim=1  device_id=0  sample_time=0.001000
      settings: SourceProductBaseCode=XP
  wires:
  c/1 -> Data Type Conversion/1
  Data Type Conversion/1 -> EtherCAT PDO Transmit 1/1, "EtherCAT PDO Transmit "/1

== system HL_control_pos_FFforce_RC_WirtualWall_Sync/High-Level Controller/Select outputs ==
  outs : Inport
  Bus Creator1 : BusCreator  Inputs=2  OutDataTypeStr=Bus: ThighForces
      settings: InheritFromInputs=off
  Bus Creator2 : BusCreator  Inputs=2  OutDataTypeStr=Bus: AllMotOut
      settings: InheritFromInputs=off
  Bus Creator3 : BusCreator  Inputs=2  OutDataTypeStr=Bus: MotOut
      settings: InheritFromInputs=off
  Bus Creator4 : BusCreator  Inputs=2  OutDataTypeStr=Bus: MotOut
      settings: InheritFromInputs=off
  Bus Creator5 : BusCreator  Inputs=2  OutDataTypeStr=Bus: AllDiskPos
      settings: InheritFromInputs=off
  Bus Selector1 : BusSelector  OutputSignals=R Leg outs.R disk mot.disk angle,L Leg outs.L disk mot.disk angle,gait,R Leg outs.rFT,L Leg outs.lFT,R Leg outs.rpos,R Leg outs.rvel,L Leg outs.lpos,L Leg outs.lvel
  disk angles : Outport
  gait out : Outport  Port=2
  FT out : Outport  Port=3
  EE mot : Outport  Port=4
  wires:
  Bus Selector1/8 -> Bus Creator4/1  "<lpos>"
  Bus Selector1/1 -> Bus Creator5/1  "<disk angle>"
  Bus Selector1/2 -> Bus Creator5/2  "<disk angle>"
  Bus Selector1/7 -> Bus Creator3/2  "<rvel>"
  Bus Selector1/4 -> Bus Creator1/1  "<rFT>"
  Bus Selector1/5 -> Bus Creator1/2  "<lFT>"
  Bus Selector1/6 -> Bus Creator3/1  "<rpos>"
  Bus Selector1/9 -> Bus Creator4/2  "<lvel>"
  Bus Creator3/1 -> Bus Creator2/1  "right"
  Bus Creator4/1 -> Bus Creator2/2  "left"
  outs/1 -> Bus Selector1/1
  Bus Creator2/1 -> EE mot/1
  Bus Creator1/1 -> FT out/1
  Bus Selector1/3 -> gait out/1  "<gait>"
  Bus Creator5/1 -> disk angles/1

== system HL_control_pos_FFforce_RC_WirtualWall_Sync/High-Level Controller/System Enable/ErrorHandling.Action.set_control_word ==
  c : Inport  OutDataTypeStr=double  PortDimensions=1
  f : TriggerPort  TriggerType=function-call  VariantControl=(inherit)  SampleTimeType=periodic  SampleTime=0.001
      settings: CopyFcn=Stateflow.SLINSF.SimulinkMan.removeBlockPreDeleteFcn  PreDeleteFcn=Stateflow.SLINSF.SimulinkMan.unsafePredeleteFcn
  Data Type Conversion : DataTypeConversion  OutDataTypeStr=uint16
  Drive1 ControlWord : xpcethercatlib/EtherCAT PDO Transmit   Priority=3  sig_name=M1 (MAXPOS).CST Mode.CST Outputs.ControlWord  sig_offset=832  sig_type=uint16  type_size=16  sig_dim=1  device_id=0  sample_time=0.001000
      settings: SourceProductBaseCode=XP
  Drive2 ControlWord : xpcethercatlib/EtherCAT PDO Transmit   Priority=3  sig_name=M2 (MAXPOS).CST Mode.CST Outputs.ControlWord  sig_offset=976  sig_type=uint16  type_size=16  sig_dim=1  device_id=0  sample_time=0.001000
      settings: SourceProductBaseCode=XP
  Drive3 ControlWord : xpcethercatlib/EtherCAT PDO Transmit   Priority=3  sig_name=M3 (MAXPOS).CST Mode.CST Outputs.ControlWord  sig_offset=1088  sig_type=uint16  type_size=16  sig_dim=1  device_id=0  sample_time=0.001000
      settings: SourceProductBaseCode=XP
  Drive4 ControlWord : xpcethercatlib/EtherCAT PDO Transmit   Priority=3  sig_name=M4 (MAXPOS).CST Mode.CST Outputs.ControlWord  sig_offset=1200  sig_type=uint16  type_size=16  sig_dim=1  device_id=0  sample_time=0.001000
      settings: SourceProductBaseCode=XP
  Drive5 ControlWord : xpcethercatlib/EtherCAT PDO Transmit   Priority=3  sig_name=M5 (MAXPOS).CST Mode.CST Outputs.ControlWord  sig_offset=1312  sig_type=uint16  type_size=16  sig_dim=1  device_id=0  sample_time=0.001000
      settings: SourceProductBaseCode=XP
  Drive6 ControlWord : xpcethercatlib/EtherCAT PDO Transmit   Priority=3  sig_name=M6 (MAXPOS).CST Mode.CST Outputs.ControlWord  sig_offset=1424  sig_type=uint16  type_size=16  sig_dim=1  device_id=0  sample_time=0.001000
      settings: SourceProductBaseCode=XP
  wires:
  c/1 -> Data Type Conversion/1
  Data Type Conversion/1 -> Drive6 ControlWord/1, Drive5 ControlWord/1, Drive4 ControlWord/1, Drive3 ControlWord/1, Drive1 ControlWord/1, Drive2 ControlWord/1

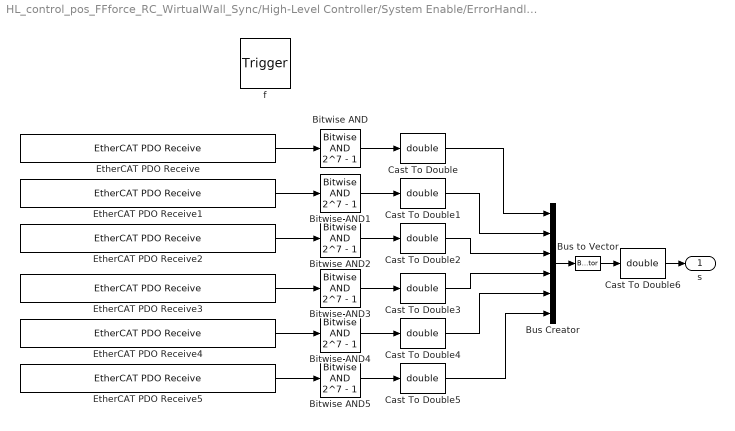
== system HL_control_pos_FFforce_RC_WirtualWall_Sync/High-Level Controller/System Enable/ErrorHandling.Device.check_status ==
  f : TriggerPort  TriggerType=function-call  VariantControl=(inherit)  SampleTimeType=periodic  SampleTime=0.001
      settings: CopyFcn=Stateflow.SLINSF.SimulinkMan.removeBlockPreDeleteFcn  PreDeleteFcn=Stateflow.SLINSF.SimulinkMan.unsafePredeleteFcn
  Bitwise AND{,1..5} (6 alike) : simulink/Logic and Bit Operations/Bitwise Operator  logicop=AND  UseBitMask=on  BitMask=2^7 - 1  BitMaskRealWorld=Stored Integer
  Bus Creator : BusCreator  Inputs=6
  Bus to Vector : BusToVector
  Cast To Double{,1..6} (7 alike) : DataTypeConversion  OutDataTypeStr=double
  EtherCAT PDO Receive : xpcethercatlib/EtherCAT PDO Receive  Priority=2  sig_name=M1 (MAXPOS).CST Mode.CST Inputs.StatusWord  sig_offset=832  sig_type=uint16  type_size=16  sig_dim=1  device_id=0  sample_time=0.001000
      settings: SourceProductBaseCode=XP
  EtherCAT PDO Receive1 : xpcethercatlib/EtherCAT PDO Receive  Priority=2  sig_name=M2 (MAXPOS).CST Mode.CST Inputs.StatusWord  sig_offset=976  sig_type=uint16  type_size=16  sig_dim=1  device_id=0  sample_time=0.001000
      settings: SourceProductBaseCode=XP
  EtherCAT PDO Receive2 : xpcethercatlib/EtherCAT PDO Receive  Priority=2  sig_name=M3 (MAXPOS).CST Mode.CST Inputs.StatusWord  sig_offset=1088  sig_type=uint16  type_size=16  sig_dim=1  device_id=0  sample_time=0.001000
      settings: SourceProductBaseCode=XP
  EtherCAT PDO Receive3 : xpcethercatlib/EtherCAT PDO Receive  Priority=2  sig_name=M4 (MAXPOS).CST Mode.CST Inputs.StatusWord  sig_offset=1200  sig_type=uint16  type_size=16  sig_dim=1  device_id=0  sample_time=0.001000
      settings: SourceProductBaseCode=XP
  EtherCAT PDO Receive4 : xpcethercatlib/EtherCAT PDO Receive  Priority=2  sig_name=M5 (MAXPOS).CST Mode.CST Inputs.StatusWord  sig_offset=1312  sig_type=uint16  type_size=16  sig_dim=1  device_id=0  sample_time=0.001000
      settings: SourceProductBaseCode=XP
  EtherCAT PDO Receive5 : xpcethercatlib/EtherCAT PDO Receive  Priority=2  sig_name=M6 (MAXPOS).CST Mode.CST Inputs.StatusWord  sig_offset=1424  sig_type=uint16  type_size=16  sig_dim=1  device_id=0  sample_time=0.001000
      settings: SourceProductBaseCode=XP
  s : Outport  OutDataTypeStr=double  PortDimensions=[6 1]
  wires:
  EtherCAT PDO Receive/1 -> Bitwise AND/1
  EtherCAT PDO Receive1/1 -> Bitwise AND1/1
  EtherCAT PDO Receive2/1 -> Bitwise AND2/1
  EtherCAT PDO Receive5/1 -> Bitwise AND5/1
  EtherCAT PDO Receive4/1 -> Bitwise AND4/1
  EtherCAT PDO Receive3/1 -> Bitwise AND3/1
  Cast To Double/1 -> Bus Creator/1
  Cast To Double1/1 -> Bus Creator/2
  Cast To Double2/1 -> Bus Creator/3
  Cast To Double3/1 -> Bus Creator/4
  Cast To Double4/1 -> Bus Creator/5
  Cast To Double5/1 -> Bus Creator/6
  Bitwise AND/1 -> Cast To Double/1
  Bitwise AND1/1 -> Cast To Double1/1
  Bitwise AND2/1 -> Cast To Double2/1
  Bitwise AND3/1 -> Cast To Double3/1
  Bitwise AND4/1 -> Cast To Double4/1
  Bitwise AND5/1 -> Cast To Double5/1
  Bus to Vector/1 -> Cast To Double6/1
  Bus Creator/1 -> Bus to Vector/1
  Cast To Double6/1 -> s/1

== system HL_control_pos_FFforce_RC_WirtualWall_Sync/High-Level Controller/System Enable/MaintainCommunication.init_ethercat ==
  note: Set Mode to
      | Torque Control
  f : TriggerPort  TriggerType=function-call  VariantControl=(inherit)  SampleTimeType=periodic  SampleTime=0.001
      settings: CopyFcn=Stateflow.SLINSF.SimulinkMan.removeBlockPreDeleteFcn  PreDeleteFcn=Stateflow.SLINSF.SimulinkMan.unsafePredeleteFcn
  Big Beckhoff : xpcethercatlib/EtherCAT Init   Priority=0  Commented=on  config_file=C:\Users\AliYasar\Desktop\AssistOnGait Simulink\Simulink Models\AssistOn-Gait-v1.4.2.xml  device_id=1  pci_bus=4  pci_slot=0  pci_function=0  initstate=2  dctuning=0  enaDebug=off  enaDC=on  errLink=off  masterDbg=off  stateChgDbg=off  baseClock=off  masterCfg=off  logFile='c:\dbglog.txt'  sample_time=0.001000  DCMode=2
      settings: SourceProductBaseCode=XP
  Constant : Constant  Value=10  OutDataTypeStr=int8
  Drive1 ModeOfOpt : xpcethercatlib/EtherCAT PDO Transmit   Priority=3  sig_name=M1 (MAXPOS).CST Mode.CST Outputs.ModeOfOperation  sig_offset=864  sig_type=int8  type_size=8  sig_dim=1  device_id=0  sample_time=0.001000
      settings: SourceProductBaseCode=XP
  Drive2 ModeOfOpt : xpcethercatlib/EtherCAT PDO Transmit   Priority=3  sig_name=M2 (MAXPOS).CST Mode.CST Outputs.ModeOfOperation  sig_offset=1008  sig_type=int8  type_size=8  sig_dim=1  device_id=0  sample_time=0.001000
      settings: SourceProductBaseCode=XP
  Drive3 ModeOfOpt : xpcethercatlib/EtherCAT PDO Transmit   Priority=3  sig_name=M3 (MAXPOS).CST Mode.CST Outputs.ModeOfOperation  sig_offset=1120  sig_type=int8  type_size=8  sig_dim=1  device_id=0  sample_time=0.001000
      settings: SourceProductBaseCode=XP
  Drive4 ModeOfOpt : xpcethercatlib/EtherCAT PDO Transmit   Priority=3  sig_name=M4 (MAXPOS).CST Mode.CST Outputs.ModeOfOperation  sig_offset=1232  sig_type=int8  type_size=8  sig_dim=1  device_id=0  sample_time=0.001000
      settings: SourceProductBaseCode=XP
  Drive5 ModeOfOpt : xpcethercatlib/EtherCAT PDO Transmit   Priority=3  sig_name=M5 (MAXPOS).CST Mode.CST Outputs.ModeOfOperation  sig_offset=1344  sig_type=int8  type_size=8  sig_dim=1  device_id=0  sample_time=0.001000
      settings: SourceProductBaseCode=XP
  Drive6 ModeOfOpt : xpcethercatlib/EtherCAT PDO Transmit   Priority=3  sig_name=M6 (MAXPOS).CST Mode.CST Outputs.ModeOfOperation  sig_offset=1456  sig_type=int8  type_size=8  sig_dim=1  device_id=0  sample_time=0.001000
      settings: SourceProductBaseCode=XP
  Small Beckhoff : xpcethercatlib/EtherCAT Init   Priority=0  config_file=C:\Users\AssistON-Gait\Desktop\AssistOnGait Simulink\Simulink Models\AssistOn-Gait-v1.4.2.xml  device_id=0  pci_bus=1  pci_slot=0  pci_function=0  initstate=2  dctuning=0  enaDebug=off  enaDC=on  errLink=off  masterDbg=off  stateChgDbg=off  baseClock=off  masterCfg=off  logFile='c:\dbglog.txt'  sample_time=0.001000  DCMode=2
      settings: SourceProductBaseCode=XP
  Terminator : Terminator
  wires:
  Small Beckhoff/1 -> Terminator/1
  Constant/1 -> Drive6 ModeOfOpt/1, Drive5 ModeOfOpt/1, Drive4 ModeOfOpt/1, Drive1 ModeOfOpt/1, Drive2 ModeOfOpt/1, Drive3 ModeOfOpt/1

== system HL_control_pos_FFforce_RC_WirtualWall_Sync/Left Leg/Jacobian Transpose [mN] -> [mN.mm//rad] ==
  states : Inport
  force [mN] : Inport  Port=2
  Bus Selector1 : BusSelector  OutputSignals=L disk mot.disk angle,L pos.s1s2s3,L pos.xytheta  OutputAsBus=on
  Bus to Vector : BusToVector
  S-Function : S-Function  FunctionName=RRP_Jacobian_Transpose  SFunctionModules='RRP_Jacobian_Transpose_wrapper'  SFunctionDeploymentMode=off  EnableBusSupport=off
  torque [mN.mm/rad] : Outport
  wires:
  states/1 -> Bus Selector1/1
  force [mN]/1 -> S-Function/2
  S-Function/1 -> torque [mN.mm/rad]/1
  Bus to Vector/1 -> S-Function/1
  Bus Selector1/1 -> Bus to Vector/1

== system HL_control_pos_FFforce_RC_WirtualWall_Sync/Left Leg/L Actuation ==
  torque [mN.mm/rad] : Inport
  M1 Target Torque : xpcethercatlib/EtherCAT PDO Transmit   Priority=3  sig_name=M4 (MAXPOS).CST Mode.CST Outputs.TargetTorque  sig_offset=1216  sig_type=int16  type_size=16  sig_dim=1  device_id=0  sample_time=0.001000
      settings: SourceProductBaseCode=XP
  M2 Target Torque : xpcethercatlib/EtherCAT PDO Transmit   Priority=3  sig_name=M5 (MAXPOS).CST Mode.CST Outputs.TargetTorque  sig_offset=1328  sig_type=int16  type_size=16  sig_dim=1  device_id=0  sample_time=0.001000
      settings: SourceProductBaseCode=XP
  M3 Target Torque : xpcethercatlib/EtherCAT PDO Transmit   Priority=3  sig_name=M6 (MAXPOS).CST Mode.CST Outputs.TargetTorque  sig_offset=1440  sig_type=int16  type_size=16  sig_dim=1  device_id=0  sample_time=0.001000
      settings: SourceProductBaseCode=XP
  Target Torque : Subsystem
  wires:
  Target Torque/3(M3_torque) -> M3 Target Torque/1
  Target Torque/2(M2_torque) -> M2 Target Torque/1
  Target Torque/1(M1_torque) -> M1 Target Torque/1
  torque [mN.mm/rad]/1 -> Target Torque/1(torque)

== system HL_control_pos_FFforce_RC_WirtualWall_Sync/Left Leg/L Outputs ==
  3RRP Forward Kinematics : AssistOn_Gait_Lib/3RRP Forward Kinematics  SystemSampleTime=-1  Latency=0  AutoFrameSizeCalculation=off
  3RRP Motion Level Kinematics : AssistOn_Gait_Lib/3RRP Motion Level Kinematics  SystemSampleTime=-1  Latency=0  AutoFrameSizeCalculation=off
  Bus Creator : BusCreator  Inputs=7
  Bus Selector1 : BusSelector  OutputSignals=disk angle
  L 3RRP : AssistOn_Gait_Lib/3RRP  SystemSampleTime=-1  Latency=0  AutoFrameSizeCalculation=off
      link override 3RRP Motor Encoder Increments/M1 Position Value: sig_name=M4 (MAXPOS).CST Mode.CST Inputs.PositionActualValue  sig_offset=1184  sig_type=int32  type_size=32  sig_dim=1
      link override 3RRP Motor Encoder Increments/M2 Position Value: sig_name=M5 (MAXPOS).CST Mode.CST Inputs.PositionActualValue  sig_offset=1296  sig_type=int32  type_size=32  sig_dim=1
      link override 3RRP Motor Encoder Increments/M3 Position Value: sig_name=M6 (MAXPOS).CST Mode.CST Inputs.PositionActualValue  sig_offset=1408  sig_type=int32  type_size=32  sig_dim=1
      link override 3RRP Motor Torque Readings/M1 Velocity Value: sig_name=M4 (MAXPOS).CST Mode.CST Inputs.TorqueActualValue  sig_offset=1280  sig_type=int16  type_size=16  sig_dim=1
      link override 3RRP Motor Torque Readings/M2 Velocity Value: sig_name=M5 (MAXPOS).CST Mode.CST Inputs.TorqueActualValue  sig_offset=1392  sig_type=int16  type_size=16  sig_dim=1
      link override 3RRP Motor Torque Readings/M3 Velocity Value: sig_name=M6 (MAXPOS).CST Mode.CST Inputs.TorqueActualValue  sig_offset=1504  sig_type=int16  type_size=16  sig_dim=1
      link override 3RRP Motor Velocity Readings/M1 Velocity Value: sig_name=M4 (MAXPOS).CST Mode.CST Inputs.Velocity Actual Value Averaged  sig_offset=1216  sig_type=int32  type_size=32  sig_dim=1
      link override 3RRP Motor Velocity Readings/M2 Velocity Value: sig_name=M5 (MAXPOS).CST Mode.CST Inputs.Velocity Actual Value Averaged  sig_offset=1328  sig_type=int32  type_size=32  sig_dim=1
      link override 3RRP Motor Velocity Readings/M3 Velocity Value: sig_name=M6 (MAXPOS).CST Mode.CST Inputs.Velocity Actual Value Averaged  sig_offset=1440  sig_type=int32  type_size=32  sig_dim=1
  L Foot : Subsystem
  L Thigh : Subsystem
  L leg outs : Outport
  wires:
  3RRP Motion Level Kinematics/1 -> Bus Creator/4  "L vel"
  Bus Creator/1 -> L leg outs/1
  3RRP Forward Kinematics/1 -> 3RRP Motion Level Kinematics/1, Bus Creator/3  "L pos"
  L Foot/1(Foot sens L) -> Bus Creator/7  "L_foot_sens"
  Bus Selector1/1 -> 3RRP Forward Kinematics/1  "<disk angle>"
  L 3RRP/2 -> 3RRP Motion Level Kinematics/2, Bus Creator/5, Bus Selector1/1  "L disk mot"
  L Thigh/1(FT vals) -> Bus Creator/6  "L_thigh_FT"
  [L_motor_T_demands] -> Bus Creator/1
  L 3RRP/1 -> Bus Creator/2  "L disk torque"

== system HL_control_pos_FFforce_RC_WirtualWall_Sync/Left Leg/Position Controller -> [mN] ==
  ref pos : Inport
  ref vel : Inport  Port=2
  estimated out : Inport  Port=3
  " " : Sum
  Bus Selector : BusSelector  OutputSignals=L pos.xytheta,L vel
  D_Controller : Subsystem
  "P_Controller\t" : Subsystem
  Control Force : Outport
  wires:
  Bus Selector/2 -> D_Controller/1(Act_Vel)  "<L vel>"
  estimated out/1 -> Bus Selector/1
  "P_Controller\t"/1(P control out) -> " "/1
  Bus Selector/1 -> "P_Controller\t"/2(Act_Pos)  "<xytheta>"
  " "/1 -> Control Force/1  "Control Force"
  D_Controller/1(D control out) -> " "/2
  ref vel/1 -> D_Controller/2(Ref_vel)
  ref pos/1 -> "P_Controller\t"/1(Ref_Pos)

== system HL_control_pos_FFforce_RC_WirtualWall_Sync/Left Leg/Subsystem ==
  L Leg Out : Inport
  Referance : Inport  Port=2
  R Referance : Inport  Port=3
  Synchronizer Controller : Subsystem
  Virtual Wall Controller : Subsystem
  Virtual Wall Control Signal : Outport
  Synchronizing Control Signal : Outport  Port=2
  wires:
  L Leg Out/1 -> Synchronizer Controller/2(L Referance), Virtual Wall Controller/1(L Leg Out)
  Referance/1 -> Virtual Wall Controller/2(Referance)
  Virtual Wall Controller/1(Virtual Wall Control Signal) -> Virtual Wall Control Signal/1
  R Referance/1 -> Synchronizer Controller/1(R Referance)
  Synchronizer Controller/1(Synchronizing Control Signal) -> Synchronizing Control Signal/1

== system HL_control_pos_FFforce_RC_WirtualWall_Sync/Left Leg/Velocity Sourced Compansator ==
  Velocity Disks : Inport
  Mode : Inport  Port=2
  DiskGains : Constant  Value=[1;1;3]
  MATLAB Function1 : MATLAB Function  TreatAsAtomicUnit=on
  Disk Forces : Outport
  wires:
  Velocity Disks/1 -> MATLAB Function1/1(Vel)
  Mode/1 -> MATLAB Function1/3(Mode)
  DiskGains/1 -> MATLAB Function1/2(MaxGain)
  MATLAB Function1/1(Torque) -> Disk Forces/1
